simulink model "basicSG1"  (R2020b)
settings: Solver=ode23tb  StartTime=0.0  StopTime=2  FixedStep=1e-3  RelTol=1e-4
undefined symbols (not defined in the file): RLOAD
libraries: powerlib x10, powerlib_extras x4, simulink x1
Description:
  | Copyright 2008-2010 The MathWorks, Inc.
settings Model: ExtModeTrigMode=oneshot  ExtModeArmWhenConnect=off  ExtModeAutoUpdateStatusClock=off  Creator=MathWorks  LastModifiedBy=talha
settings DataIOCC: InitialState=xinit  SaveFormat=Array  SignalLoggingSaveFormat=ModelDataLogs  SaveOutput=off  ReturnWorkspaceOutputs=off  TimeSaveName=t  SignalLoggingName=sigsOut
settings OptimizationCC: BooleanDataType=off  ExpressionDepthLimit=2147483647  InitFltsAndDblsToZero=on  LifeSpan=inf
settings DebuggingCC: SaveWithParameterizedLinksMsg=none  UnderspecifiedInitializationDetection=Classic  MergeDetectMultiDrivingBlocksExec=none  SignalResolutionControl=TryResolveAllWithWarning  MultiTaskDSMMsg=warning  MultiTaskCondExecSysMsg=none  SigSpecEnsureSampleTimeMsg=none  FcnCallInpInsideContextMsg=warning  SignalLabelMismatchMsg=warning  StateNameClashWarn=warning  SFUnexpectedBacktrackingDiag=warning  SFNoUnconditionalDefaultTransitionDiag=warning  SFExecutionAtInitializationDiag=none  ArithmeticOperatorsInVariantConditions=warning
settings HardwareCC: ProdBitPerPointer=32  ProdBitPerSizeT=32  ProdBitPerPtrDiffT=32  ProdLargestAtomicFloat=None  ProdIntDivRoundTo=Undefined  ProdEndianess=Unspecified  ProdWordSize=32  ProdHWDeviceType=32-bit Generic  TargetUnknown=on
settings ModelReferenceCC: PropagateSignalLabelsOutOfModel=off
settings SFSimCC: SimUseLocalCustomCode=off  CustomCodeUndefinedFunction=UseInterfaceOnly
settings RTWCC: RTWUseLocalCustomCode=off
settings CodeAppCC: StateflowObjectComments=on
settings GRTTargetCC: TargetFcnLib=ansi_tfl_tmw.mat  TargetLangStandard=C89/C90 (ANSI)  CombineOutputUpdateFcns=off  GRTInterface=on
settings ConfigComp: CovMetricSettings=dw  CovSaveCumulativeToWorkspaceVar=on  CovSaveSingleToWorkspaceVar=on  CovExternalEMLEnable=off  CovSFcnEnable=off
settings SimscapeCC: SimscapeNormalizeSystem=off

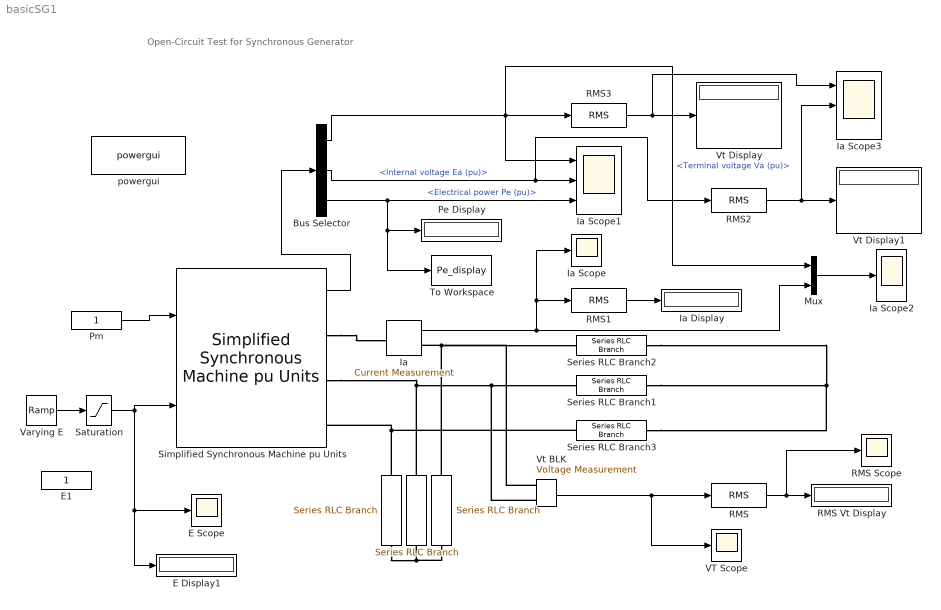
== system basicSG1 ==
  note: Open-Circuit Test for Synchronous Generator
  " " : powerlib/Elements/Series RLC Branch  LConnTagsString=__new0  RConnTagsString=__new0  BranchType=R  Resistance=36e4  Inductance=5e-3*5  SetiL0=off  InitialCurrent=0.1  Capacitance=1e-6  Setx0=off  InitialVoltage=0  Measurements=Branch voltage and current
  " " : powerlib/Elements/Series RLC Branch  LConnTagsString=__new0  RConnTagsString=__new0  BranchType=R  Resistance=36e4  Inductance=5e-3*5  SetiL0=off  InitialCurrent=0.1  Capacitance=1e-6  Setx0=off  InitialVoltage=0  Measurements=Branch voltage and current
  " " : powerlib/Elements/Series RLC Branch  LConnTagsString=__new0  RConnTagsString=__new0  BranchType=R  Resistance=36e4  Inductance=5e-3*5  SetiL0=off  InitialCurrent=0.1  Capacitance=1e-6  Setx0=off  InitialVoltage=0  Measurements=Branch voltage and current
  Bus Selector : BusSelector  OutputSignals=Terminal voltage Va (pu),Internal voltage Ea (pu),Electrical power Pe (pu)
  E Display1 : Display
  E Scope : Scope
  E1 : Constant
  Ia : powerlib/Measurements/Current Measurement  Tag=PoWeRsYsTeMmEaSuReMeNt  PhasorSimulation=off  OutputType=Magnitude  PSBequivalent=0
  Ia Display : Display
  Ia Scope : Scope
  Ia Scope1 : Scope  NumInputPorts=3
  Ia Scope2 : Scope
  Ia Scope3 : Scope  NumInputPorts=3
  Mux : Mux  Inputs=2
  Pe Display : Display
  Pm : Constant
  RMS{,1..3} (4 alike) : powerlib_extras/Measurements/RMS  f1=50
      settings: SourceProductBaseCode=PS
  RMS Scope : Scope
  RMS Vt Display : Display
  Saturation : Saturate  UpperLimit=1.7  LowerLimit=0
  Series RLC Branch1 : powerlib/Elements/Series RLC Branch  LConnTagsString=__new0  RConnTagsString=__new0  BranchType=R  Resistance=RLOAD  Inductance=5e-3*5  SetiL0=off  InitialCurrent=0.1  Capacitance=1e-6  Setx0=off  InitialVoltage=0  Measurements=Branch voltage and current
  Series RLC Branch2 : powerlib/Elements/Series RLC Branch  LConnTagsString=__new0  RConnTagsString=__new0  BranchType=R  Resistance=RLOAD  Inductance=5e-3*5  SetiL0=off  InitialCurrent=0.1  Capacitance=1e-6  Setx0=off  InitialVoltage=0  Measurements=Branch voltage and current
  Series RLC Branch3 : powerlib/Elements/Series RLC Branch  LConnTagsString=__new0  RConnTagsString=__new0  BranchType=R  Resistance=RLOAD  Inductance=5e-3*5  SetiL0=off  InitialCurrent=0.1  Capacitance=1e-6  Setx0=off  InitialVoltage=0  Measurements=Branch voltage and current
  Simplified Synchronous Machine pu Units : powerlib/Machines/Simplified Synchronous Machine pu Units  ConnectionType=3-wire Y  MechanicalLoad=Mechanical power Pm  MeasurementBus=off  NominalParameters=[1000 220 50]  Mechanical=[0.5 0.5 2]  InternalRL="[0.1  1]"  InitialConditions="[ 0,0   0,0,0   0,0,0 ]"  IterativeDiscreteModel=Trapezoidal non iterative  TsBlock=-1  TsPowergui=0  LoadFlowParameters=[1,0,0,0,0]  Units=0  BusType=PV  Pref=0  Qref=0  Qmin=-inf  Qmax=+inf  PLF=0  QLF=0
      settings: SourceProductBaseCode=PS
  To Workspace : ToWorkspace  VariableName=Pe_display  SaveFormat=Timeseries  SampleTime=-1
      settings: Decimation=20
  VT Scope : Scope
  Varying E : simulink/Sources/Ramp  slope=1  start=0  InitialOutput=0
  Vt BLK : powerlib/Measurements/Voltage Measurement  PhasorSimulation=off  OutputType=Complex  PSBequivalent=0
  Vt Display : Display
  Vt Display1 : Display
  powergui : powerlib/powergui  Priority=2  SimulationMode=Continuous  SampleTime=0  frequency=60  Iterations=50  frequencyindice=50  Pbase=100e6  ErrMax=1e-4  UnitsV=kV  UnitsW=MW  buscounter=0  FunctionMessages=off  echomessages=off  EnableUseOfTLC=off  CurrentSourceSwitches=off  DisableSnubberDevices=off  DisableRonSwitches=off  DisableVfSwitches=off  DisplayEquations=off  AutomaticDiscreteSolvers=off  SolverType=Tustin  Interpol=off  ExternalGateDelay=off  methode=off  Ts=0  x0status=blocks  SPID=off  SwTol=0  HookPort=off  NonlinearTolerance=1e-4  nMaxIteration=100  ContinueOnMaxIteration=off  RestoreLinks=warning  ResistiveCurrentMeasurement=off  Frange=[0:2:500]  Ylog=off  Xlog=off  ShowGrid=off  save=off  variable=ZData  structure=0  ZoomFFT=on  StartTime=0.0  cycles=1  DisplayStyle=off  fundamental=60  FreqAxis=off  MaxFrequency=1000  frequencyindicesteady=1  RmsSteady=1  display=off
  wires:
  Pm/1 -> Simplified Synchronous Machine pu Units/1
  Ia/1 -> Mux/2, RMS1/1, Ia Scope/1
  RMS1/1 -> Ia Display/1
  RMS/1 -> RMS Vt Display/1, RMS Scope/1
  Vt BLK/1 -> VT Scope/1, RMS/1
  Simplified Synchronous Machine pu Units/1 -> Bus Selector/1
  RMS3/1 -> Ia Scope3/1, Vt Display/1
  Varying E/1 -> Saturation/1
  Bus Selector/3 -> Ia Scope1/3, Pe Display/1, To Workspace/1  "<Electrical power Pe (pu)>"
  Bus Selector/1 -> RMS3/1, Ia Scope1/1, Mux/1  "<Terminal voltage Va (pu)>"
  Bus Selector/2 -> RMS2/1, Ia Scope1/2  "<Internal voltage Ea (pu)>"
  RMS2/1 -> Ia Scope3/2, Vt Display1/1
  Mux/1 -> Ia Scope2/1
  Saturation/1 -> E Display1/1, E Scope/1, Simplified Synchronous Machine pu Units/2
  connections:
  Simplified Synchronous Machine pu Units/RConn1 -- Ia/LConn1
  Vt BLK/LConn1 -- Series RLC Branch2/LConn1 -- " "/LConn1 -- Ia/RConn1
  Simplified Synchronous Machine pu Units/RConn2 -- " "/LConn1 -- Vt BLK/LConn2 -- Series RLC Branch1/LConn1
  " "/LConn1 -- Simplified Synchronous Machine pu Units/RConn3 -- Series RLC Branch3/LConn1
  Series RLC Branch2/RConn1 -- Series RLC Branch3/RConn1 -- Series RLC Branch1/RConn1
  " "/RConn1 -- ?
